simulink model "SIMrun_LIP"  (R2024b)
settings: Solver=FixedStepDiscrete  StartTime=0.0  StopTime=50  FixedStep=Ts  RelTol=1e-3
values from neighbouring files (symbols this model uses):
  a = 1    [LIP_main.m]
  b = 1    [LIP_main.m]
  CT = cosh(Ts/Tc)    [LIP_main.m]
  ST = sinh(Ts/Tc)    [LIP_main.m]
  Tc = sqrt(z0/g)    [LIP_main.m]
  Ts = 0.2    [H_LIP_main_analytical.m]    (also in H_LIP_main_ode45_solver.m; LIP_main.m = 0.35)
  vd = 1    [LIP_main.m]
  xd = [-0.1;1]    [H_LIP_main_analytical.m]    (also in H_LIP_main_ode45_solver.m; LIP_main.m = 0.1)
  xf_i = -0.05    [LIP_main.m]
settings Model: Creator=FurusTM  LastModifiedBy=FurusTM

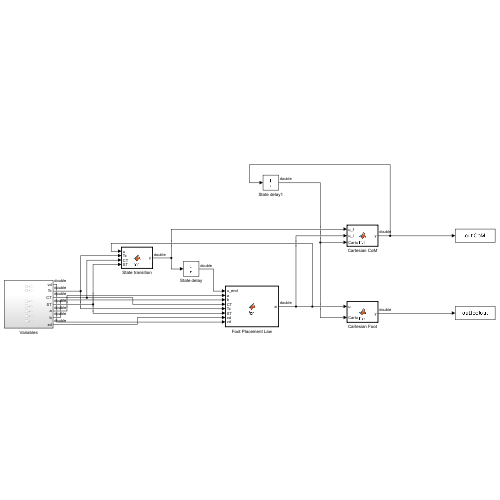
[thumbnail: Simulink's stored preview of the top-level diagram]
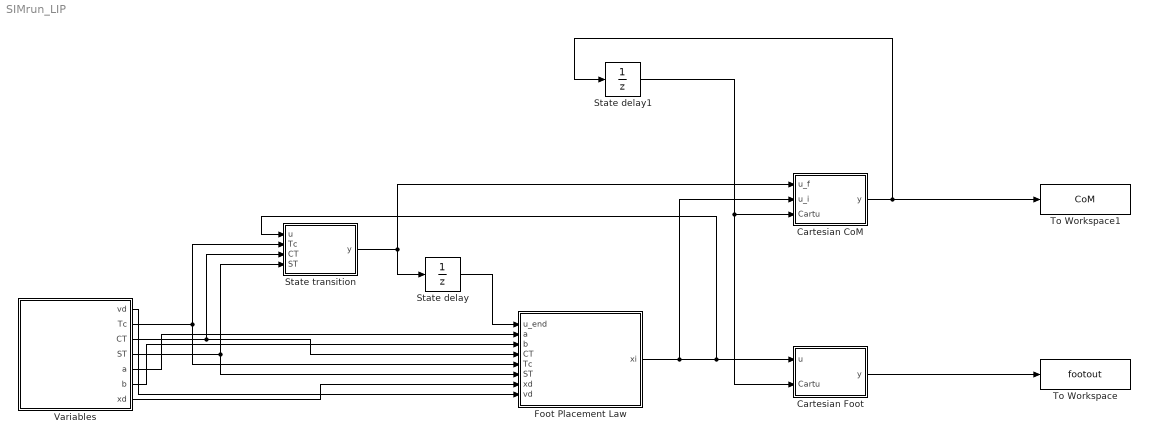
== system SIMrun_LIP ==
  Cartesian CoM : MATLAB Function  TreatAsAtomicUnit=on
  Cartesian Foot : MATLAB Function  TreatAsAtomicUnit=on
  Foot Placement Law : MATLAB Function  TreatAsAtomicUnit=on
  State delay : UnitDelay  InitialCondition=[0.2+xf_i;vd]  SampleTime=Ts  HasFrameUpgradeWarning=on
  State delay1 : UnitDelay  InitialCondition=0.2+xf_i  SampleTime=Ts  HasFrameUpgradeWarning=on
  State transition : MATLAB Function  TreatAsAtomicUnit=on
  To Workspace : ToWorkspace  VariableName=footout  SaveFormat=Timeseries  SampleTime=-1
  To Workspace1 : ToWorkspace  VariableName=CoM  SaveFormat=Timeseries  SampleTime=-1
  Variables : Subsystem
  wires:
  State transition/1(y) -> State delay/1, Cartesian CoM/1(u_f)
  Foot Placement Law/1(xi) -> Cartesian CoM/2(u_i), State transition/1(u), Cartesian Foot/1(u)
  Variables/2(Tc) -> State transition/2(Tc), Foot Placement Law/5(Tc)
  Variables/3(CT) -> State transition/3(CT), Foot Placement Law/4(CT)
  Variables/4(ST) -> State transition/4(ST), Foot Placement Law/6(ST)
  Variables/5(a) -> Foot Placement Law/2(a)
  Variables/6(b) -> Foot Placement Law/3(b)
  Variables/1(vd) -> Foot Placement Law/8(vd)
  Variables/7(xd) -> Foot Placement Law/7(xd)
  Cartesian CoM/1(y) -> State delay1/1, To Workspace1/1
  State delay1/1 -> Cartesian Foot/2(Cartu), Cartesian CoM/3(Cartu)
  Cartesian Foot/1(y) -> To Workspace/1
  State delay/1 -> Foot Placement Law/1(u_end)

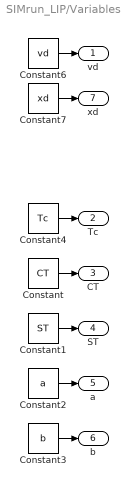
== system SIMrun_LIP/Variables ==
  Constant : Constant  Value=CT
  Constant1 : Constant  Value=ST
  Constant2 : Constant  Value=a
  Constant3 : Constant  Value=b
  Constant4 : Constant  Value=Tc
  Constant6 : Constant  Value=vd
  Constant7 : Constant  Value=xd
  vd : Outport
  Tc : Outport  Port=2
  CT : Outport  Port=3
  ST : Outport  Port=4
  a : Outport  Port=5
  b : Outport  Port=6
  xd : Outport  Port=7
  wires:
  Constant3/1 -> b/1
  Constant/1 -> CT/1
  Constant1/1 -> ST/1
  Constant4/1 -> Tc/1
  Constant6/1 -> vd/1
  Constant2/1 -> a/1
  Constant7/1 -> xd/1

== matlab function SIMrun_LIP/State transition ==
  data: u input; y output; Tc input; CT input; ST input
function y = fcn(u,Tc,CT,ST)
% state transition matrix
A = [CT,Tc*ST;
     ST/Tc,CT];

y = A * u;

== matlab function SIMrun_LIP/Foot Placement Law ==
  data: u_end input; xi output; a input; b input; CT input; Tc input; ST input; xd input; vd input
function xi = fcn(u_end,a,b,CT,Tc,ST,xd,vd)

%foot placement from intial COM
xi = [(a*CT*(xd - ST*Tc*vd) + b*(ST/Tc)*(vd - CT*u_end(2))) / (a*CT^2 + b*(ST/Tc)^2); u_end(2)];

== matlab function SIMrun_LIP/Cartesian Foot ==
  data: u input; y output; Cartu input
function y = fcn(u,Cartu)

y = - u(1) + Cartu;

== matlab function SIMrun_LIP/Cartesian CoM ==
  data: u_f input; u_i input; y output; Cartu input
function y = fcn(u_f,u_i,Cartu)

y = u_f(1) + Cartu - u_i(1);
